simulink model "A_DIOL_BicopterControl"  (R2022a)
settings: Solver=FixedStepAuto  StartTime=0.0  StopTime=110  FixedStep=1e-4  RelTol=1e-3
values from neighbouring files (symbols this model uses):
  k = place(A,B,p)    [A_DIOL_runner.m]    (also in A_DIOL_sim_runner.m; print_DE_FL.m)
undefined symbols (not defined in the file or in its folder): sigbuilder_block
libraries: spsFirstOrderFilterLib x6
settings Model: Creator=PhDstudent1  LastModifiedBy=NITRO5

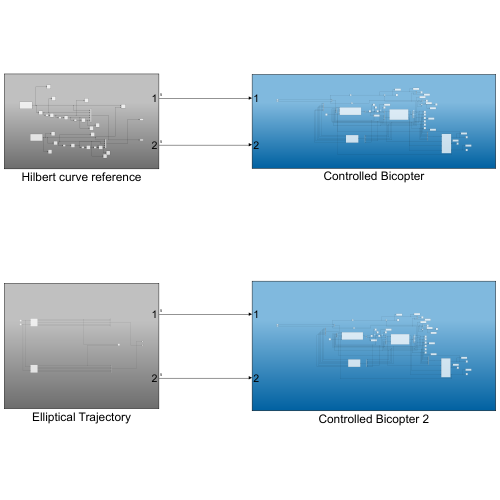
[thumbnail: Simulink's stored preview of the top-level diagram]
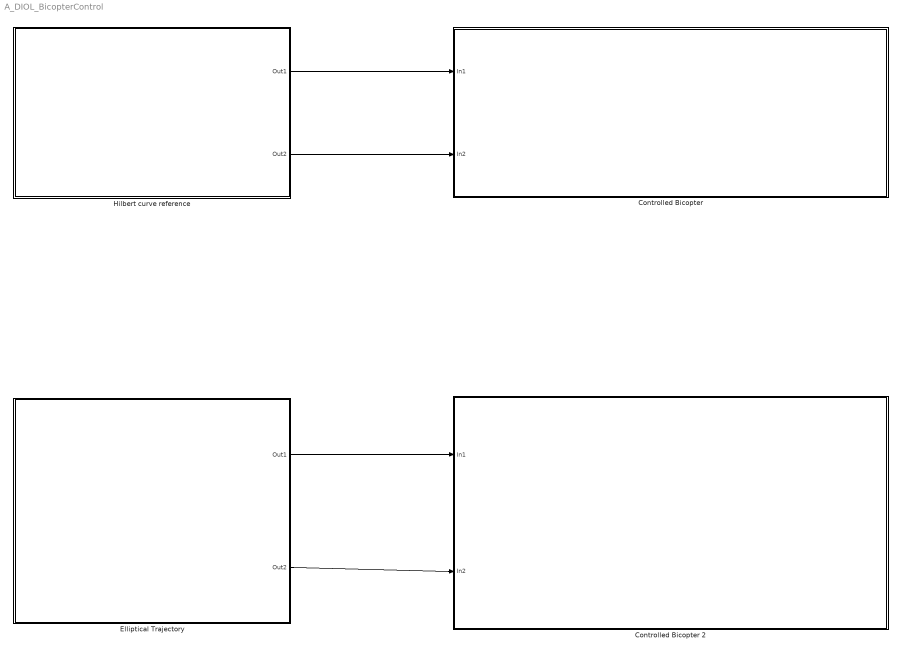
== system A_DIOL_BicopterControl ==
  Controlled Bicopter : Subsystem
  Controlled Bicopter 2 : Subsystem
  Elliptical Trajectory : Subsystem
  Hilbert curve reference : Subsystem
  wires:
  Hilbert curve reference/1(Out1) -> Controlled Bicopter/1(In1)
  Hilbert curve reference/2(Out2) -> Controlled Bicopter/2(In2)
  Elliptical Trajectory/1(Out1) -> Controlled Bicopter 2/1(In1)
  Elliptical Trajectory/2(Out2) -> Controlled Bicopter 2/2(In2)

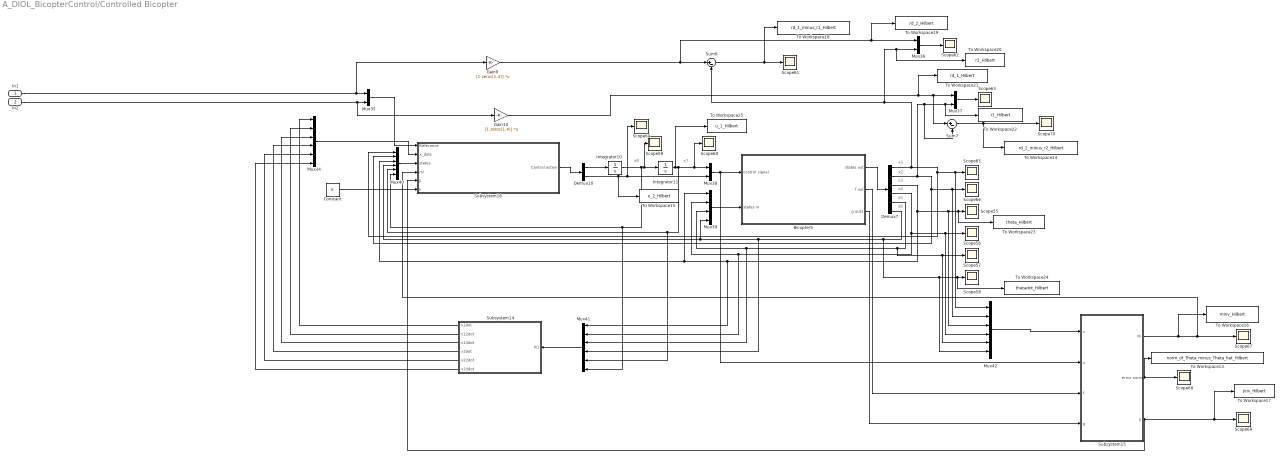
== system A_DIOL_BicopterControl/Controlled Bicopter ==
  note: x4
  note: x1
  note: x8
  note: x5
  note: x6
  note: x7
  note: x2
  note: x3
  In1 : Inport
  In2 : Inport  Port=2
  Bicopter5 : Subsystem
  Constant : Constant  Value=k
  Demux10 : Demux  Outputs=2
  Demux7 : Demux  Outputs=6
  Gain10 : Gain  Gain=[1 zeros(1,4)]  Multiplication=Matrix(K*u)
  Gain9 : Gain  Gain=[1 zeros(1,4)]  Multiplication=Matrix(K*u)
  Integrator10 : Integrator  InitialCondition=2
  Integrator11 : Integrator  InitialCondition=15
  Mux{34,40..42} (4 alike) : Mux  Inputs=6
  Mux{35..38} (4 alike) : Mux  Inputs=2
  Mux39 : Mux
  Scope{55..70} (16 alike) : Scope
  Subsystem14 : Subsystem
  Subsystem15 : Subsystem
  Subsystem16 : Subsystem
  Sum6 : Sum  Inputs=|+-
  Sum7 : Sum  Inputs=|+-
  To Workspace13 : ToWorkspace  VariableName=norm_of_Theta_minus_Theta_hat_Hilbert  SaveFormat=Timeseries  SampleTime=-1
  To Workspace14 : ToWorkspace  VariableName=rd_2_minus_r2_Hilbert  SaveFormat=Timeseries  SampleTime=-1
  To Workspace15 : ToWorkspace  VariableName=u_2_Hilbert  SaveFormat=Timeseries  SampleTime=-1
  To Workspace16 : ToWorkspace  VariableName=minv_Hilbert  SaveFormat=Timeseries  SampleTime=-1
  To Workspace17 : ToWorkspace  VariableName=Jinv_Hilbert  SaveFormat=Timeseries  SampleTime=-1
  To Workspace18 : ToWorkspace  VariableName=rd_1_minus_r1_Hilbert  SaveFormat=Timeseries  SampleTime=-1
  To Workspace19 : ToWorkspace  VariableName=rd_2_Hilbert  SaveFormat=Timeseries  SampleTime=-1
  To Workspace20 : ToWorkspace  VariableName=r2_Hilbert  SaveFormat=Timeseries  SampleTime=-1
  To Workspace21 : ToWorkspace  VariableName=rd_1_Hilbert  SaveFormat=Timeseries  SampleTime=-1
  To Workspace22 : ToWorkspace  VariableName=r1_Hilbert  SaveFormat=Timeseries  SampleTime=-1
  To Workspace23 : ToWorkspace  VariableName=theta_Hilbert  SaveFormat=Timeseries  SampleTime=-1
  To Workspace24 : ToWorkspace  VariableName=thetadot_Hilbert  SaveFormat=Timeseries  SampleTime=-1
  To Workspace25 : ToWorkspace  VariableName=u_1_Hilbert  SaveFormat=Timeseries  SampleTime=-1
  wires:
  Sum7/1 -> To Workspace14/1, Scope70/1
  Bicopter5/2(f out) -> Subsystem15/3(f)
  Demux7/6 -> Mux42/6, To Workspace24/1, Scope58/1, Mux41/4, Mux39/4, Mux40/4
  Demux7/2 -> Sum7/2, To Workspace22/1, Mux37/2, Mux42/2, Scope66/1, Mux40/2
  Demux7/1 -> To Workspace20/1, Mux36/2, Sum6/2, Mux42/1, Scope65/1, Mux40/1
  Subsystem14/6(x23dot) -> Mux34/6
  Demux7/4 -> Mux42/4, Scope56/1, Mux41/2, Mux39/2
  Bicopter5/1(states out) -> Demux7/1
  Integrator10/1 -> Mux41/6, Mux40/6, Scope59/1, Integrator11/1
  Mux42/1 -> Subsystem15/1(x)
  Subsystem15/2(error norm) -> To Workspace13/1, Scope68/1
  Demux7/5 -> Mux41/3, Mux39/3, Mux42/5, Scope57/1
  Mux39/1 -> Bicopter5/2(states in)
  Subsystem15/1(mi) -> To Workspace16/1, Scope67/1, Subsystem16/4(mi)
  Subsystem14/4(x2dot) -> Mux34/4
  Subsystem14/1(x1dot) -> Mux34/1
  Integrator11/1 -> To Workspace25/1, Mux41/5, Mux40/5, Scope60/1, Mux38/1
  Bicopter5/3(g out1) -> Subsystem15/4(g)
  Demux10/2 -> To Workspace15/1, Scope64/1, Mux38/2
  In2/1 -> Gain10/1, Mux35/2
  Gain9/1 -> To Workspace19/1, Mux36/1, Sum6/1
  Demux10/1 -> Integrator10/1
  Mux40/1 -> Subsystem16/3(states)
  In1/1 -> Gain9/1, Mux35/1
  Mux37/1 -> Scope63/1
  Subsystem15/3(Ji) -> Subsystem16/5(Ji), To Workspace17/1, Scope69/1
  Mux34/1 -> Subsystem16/2(x_dots)
  Subsystem16/1(Control action) -> Demux10/1
  Mux35/1 -> Subsystem16/1(Reference)
  Sum6/1 -> To Workspace18/1, Scope61/1
  Constant/1 -> Subsystem16/6(k)
  Subsystem14/2(x12dot) -> Mux34/2
  Gain10/1 -> To Workspace21/1, Sum7/1, Mux37/1
  Mux38/1 -> Subsystem15/2(u), Bicopter5/1(control signal)
  Demux7/3 -> Mux42/3, To Workspace23/1, Scope55/1, Mux41/1, Mux39/1, Mux40/3
  Mux41/1 -> Subsystem14/1(In1)
  Subsystem14/3(x13dot) -> Mux34/3
  Subsystem14/5(x22dot) -> Mux34/5
  Mux36/1 -> Scope62/1

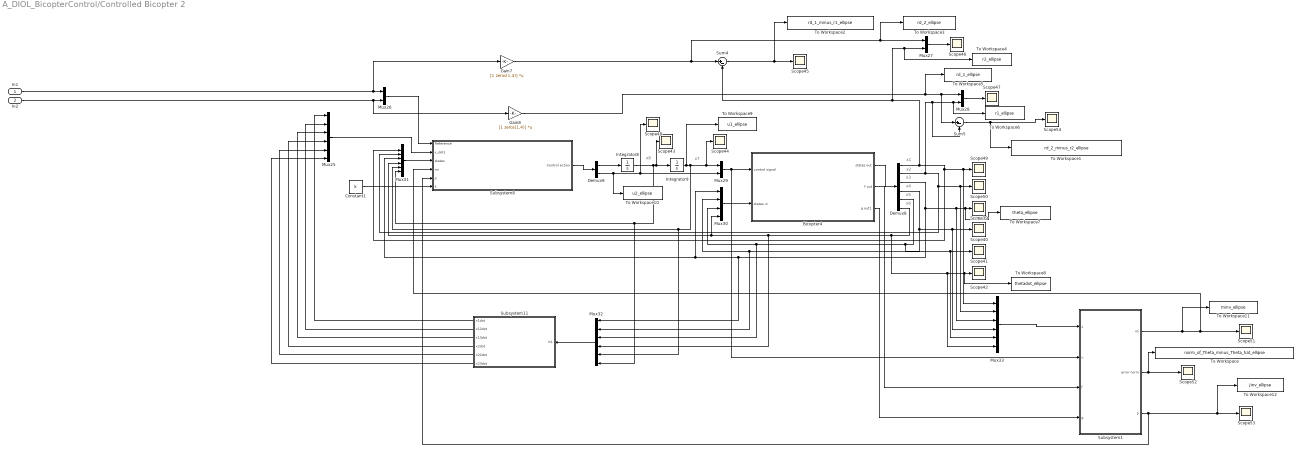
== system A_DIOL_BicopterControl/Controlled Bicopter 2 ==
  note: x4
  note: x1
  note: x8
  note: x6
  note: x5
  note: x7
  note: x3
  note: x2
  In1 : Inport
  In2 : Inport  Port=2
  Bicopter4 : Subsystem
  Constant1 : Constant  Value=k
  Demux8 : Demux  Outputs=6
  Demux9 : Demux  Outputs=2
  Gain7 : Gain  Gain=[1 zeros(1,4)]  Multiplication=Matrix(K*u)
  Gain8 : Gain  Gain=[1 zeros(1,4)]  Multiplication=Matrix(K*u)
  Integrator8 : Integrator
  Integrator9 : Integrator  InitialCondition=10
  Mux{25,31..33} (4 alike) : Mux  Inputs=6
  Mux{26..29} (4 alike) : Mux  Inputs=2
  Mux30 : Mux
  Scope{39..54} (16 alike) : Scope
  Subsystem1 : Subsystem
  Subsystem11 : Subsystem
  Subsystem8 : Subsystem
  Sum4 : Sum  Inputs=|+-
  Sum5 : Sum  Inputs=|+-
  To Workspace : ToWorkspace  VariableName=norm_of_Theta_minus_Theta_hat_ellipse  SaveFormat=Timeseries  SampleTime=-1
  To Workspace1 : ToWorkspace  VariableName=rd_2_minus_r2_ellipse  SaveFormat=Timeseries  SampleTime=-1
  To Workspace10 : ToWorkspace  VariableName=u2_ellipse  SaveFormat=Timeseries  SampleTime=-1
  To Workspace11 : ToWorkspace  VariableName=minv_ellipse  SaveFormat=Timeseries  SampleTime=-1
  To Workspace12 : ToWorkspace  VariableName=Jinv_ellipse  SaveFormat=Timeseries  SampleTime=-1
  To Workspace2 : ToWorkspace  VariableName=rd_1_minus_r1_ellipse  SaveFormat=Timeseries  SampleTime=-1
  To Workspace3 : ToWorkspace  VariableName=rd_2_ellipse  SaveFormat=Timeseries  SampleTime=-1
  To Workspace4 : ToWorkspace  VariableName=r2_ellipse  SaveFormat=Timeseries  SampleTime=-1
  To Workspace5 : ToWorkspace  VariableName=rd_1_ellipse  SaveFormat=Timeseries  SampleTime=-1
  To Workspace6 : ToWorkspace  VariableName=r1_ellipse  SaveFormat=Timeseries  SampleTime=-1
  To Workspace7 : ToWorkspace  VariableName=theta_ellipse  SaveFormat=Timeseries  SampleTime=-1
  To Workspace8 : ToWorkspace  VariableName=thetadot_ellipse  SaveFormat=Timeseries  SampleTime=-1
  To Workspace9 : ToWorkspace  VariableName=u1_ellipse  SaveFormat=Timeseries  SampleTime=-1
  wires:
  Subsystem11/2(x12dot) -> Mux25/2
  Demux8/6 -> Mux33/6, To Workspace8/1, Scope42/1, Mux32/4, Mux30/4, Mux31/4
  Subsystem1/3(Ji) -> To Workspace12/1, Scope53/1, Subsystem8/5(Ji)
  Integrator8/1 -> Mux32/6, Mux31/6, Scope43/1, Integrator9/1
  Subsystem11/6(x23dot) -> Mux25/6
  Demux8/4 -> Mux33/4, Scope40/1, Mux32/2, Mux30/2
  Integrator9/1 -> To Workspace9/1, Mux32/5, Mux31/5, Scope44/1, Mux29/1
  Demux8/1 -> To Workspace4/1, Mux27/2, Sum4/2, Mux33/1, Scope49/1, Mux31/1
  Subsystem1/1(mi) -> To Workspace11/1, Scope51/1, Subsystem8/4(mi)
  In1/1 -> Gain7/1, Mux26/1
  Demux8/2 -> Sum5/2, To Workspace6/1, Mux28/2, Mux33/2, Scope50/1, Mux31/2
  Subsystem8/1(Control action) -> Demux9/1
  Constant1/1 -> Subsystem8/6(k)
  Demux8/5 -> Mux32/3, Mux30/3, Mux33/5, Scope41/1
  Bicopter4/2(f out) -> Subsystem1/3(f)
  Subsystem11/5(x22dot) -> Mux25/5
  Subsystem11/3(x13dot) -> Mux25/3
  Mux27/1 -> Scope46/1
  Subsystem11/4(x2dot) -> Mux25/4
  Demux9/2 -> To Workspace10/1, Scope48/1, Mux29/2
  Demux9/1 -> Integrator8/1
  Mux26/1 -> Subsystem8/1(Reference)
  Mux30/1 -> Bicopter4/2(states in)
  Demux8/3 -> Mux33/3, To Workspace7/1, Scope39/1, Mux32/1, Mux30/1, Mux31/3
  Mux25/1 -> Subsystem8/2(x_dots)
  Gain7/1 -> To Workspace3/1, Mux27/1, Sum4/1
  Mux31/1 -> Subsystem8/3(states)
  Bicopter4/3(g out1) -> Subsystem1/4(g)
  Mux33/1 -> Subsystem1/1(x)
  Subsystem1/2(error norm) -> To Workspace/1, Scope52/1
  Mux29/1 -> Subsystem1/2(u), Bicopter4/1(control signal)
  Sum4/1 -> To Workspace2/1, Scope45/1
  Mux28/1 -> Scope47/1
  Mux32/1 -> Subsystem11/1(In1)
  Subsystem11/1(x1dot) -> Mux25/1
  Sum5/1 -> To Workspace1/1, Scope54/1
  In2/1 -> Gain8/1, Mux26/2
  Gain8/1 -> To Workspace5/1, Sum5/1, Mux28/1
  Bicopter4/1(states out) -> Demux8/1

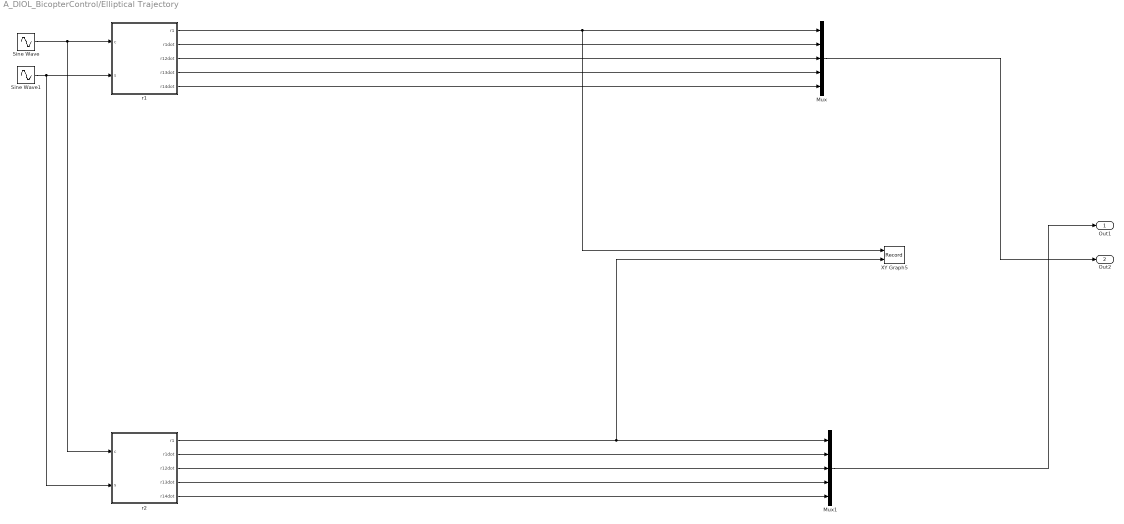
== system A_DIOL_BicopterControl/Elliptical Trajectory ==
  Mux : Mux  Inputs=5
  Mux1 : Mux  Inputs=5
  Sine Wave : Sin  Phase=pi/2  SampleTime=0
  Sine Wave1 : Sin  SampleTime=0
  XY Graph5 : Record  FileSettingsInternal="{\"entries\":[{\"content\":{\"excelSettings\":{\"content\":{},\"type\":\"Streamout.ExcelSettings\"}},\"type\":\"Streamout.FileSettingStorage\",\"uuid\":\"26a49ed7-52eb-4951-809f-6988e8d13940\"}],\"packageUris\":[\"http://schema.mathworks.com/mf0/streamout_blocks/R2020a\"],\"version\":\"1.0\"}"  Layout=[1 1]  SignalsInternal="{\"entries\":[{\"content\":{\"signals\":[{\"content\":{\"blockPath\":[\"DE_IOL/Elliptical Trajectory/XY Graph5\"],\"channel\":[],\"dimensions\":[1],\"domain\":\"DE_IOL/Elliptical Trajectory/XY Graph5\",\"lineColor\":\"#0072bd\",\"plots\":[],\"port\":1,\"sid\":[],\"signalID\":8873,\"signalName\":\"r1:1\"},\"type\":\"RecordBlkView.Signal\",\"uuid\":\"5bdcea52-0e7e-48eb-8d84-bb9175bf30af\"},{\"content\":{\"blockPath\":[\"DE_IOL/Elliptical Trajectory/XY Graph5\"],\"channel\":[],\"dimensions\":[1],\"domain\":\"DE_IOL/Elliptical Trajectory/XY Graph5\",\"lineColor\":\"#d95319\",\"plots\":[],\"port\":2,\"sid\":[],\"signalID\":8876,\"signalName\":\"r2:1\"},\"type\":\"RecordBlkView.Signal\",\"uuid\":\"504f0850-e16c-4121-9ee7-25123b3e2c1d\"}]},\"type\":\"RecordBlkView.InputSignals\",\"uuid\":\"3da81941-7f27-4a40-ba46-ff9135730fe0\"}],\"packageUris\":[\"http://schema.mathworks.com/mf0/streamout_blocks/R2020a\"],\"version\":\"1.0\"}"  VisualizationBindings="{\"xyplotplugin\":{\"info\":[{\"series\":[],\"subplotID\":1}]}}"  CompatibilityTag=XY
  r1 : MATLAB Function  TreatAsAtomicUnit=on
  r2 : MATLAB Function  TreatAsAtomicUnit=on
  Out1 : Outport
  Out2 : Outport  Port=2
  wires:
  Mux/1 -> Out2/1
  Mux1/1 -> Out1/1
  Sine Wave/1 -> r2/1(c), r1/1(c)
  Sine Wave1/1 -> r2/2(s), r1/2(s)
  r1/1(r1) -> XY Graph5/1, Mux/1
  r1/2(r1dot) -> Mux/2
  r1/3(r12dot) -> Mux/3
  r1/4(r13dot) -> Mux/4
  r1/5(r14dot) -> Mux/5
  r2/1(r1) -> XY Graph5/2, Mux1/1
  r2/2(r1dot) -> Mux1/2
  r2/3(r12dot) -> Mux1/3
  r2/4(r13dot) -> Mux1/4
  r2/5(r14dot) -> Mux1/5

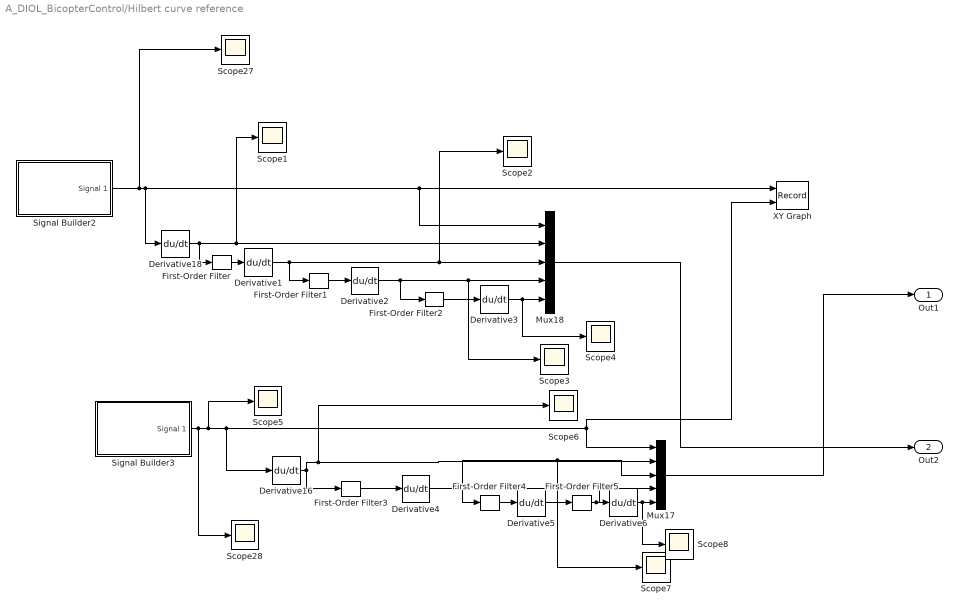
== system A_DIOL_BicopterControl/Hilbert curve reference ==
  Derivative{1..6,16,18} (8 alike) : Derivative
  First-Order Filter{,1..5} (6 alike) : spsFirstOrderFilterLib/First-Order Filter  FilterType=Lowpass  Tc=5e-01  Ts=0  Initialize=on  Vac_Init=[0, 0, 60]  Vdc_Init=0  PlotResponse=off  FreqRange="[0,  200,  1]"
  Mux17 : Mux  Inputs=5
  Mux18 : Mux  Inputs=5
  Scope{1..8,27..28} (10 alike) : Scope
  Signal Builder2 : Subsystem  Tag=STV Subsys  LoadFcn=sigbuilder_block('load');  StartFcn=sigbuilder_block('start');  StopFcn=sigbuilder_block('stop');  ClipboardFcn=sigbuilder_block('clipboard');  mask(Sigbuilder block){tuvar=[0:10]}
      mask help: Simulink:masks:SigbuilderBlock_MD
      mask init:
      | if ~strcmp(get_param(bdroot(gcbh),'SimulationStatus'),'stopped') tuvar = sigbuilder_block('maskInit'); end
      settings: CopyFcn=sigbuilder_block('copy');  DeleteFcn=sigbuilder_block('delete');  ModelCloseFcn=sigbuilder_block('modelClose');  PreSaveFcn=sigbuilder_block('preSave');  PauseFcn=sigbuilder_block('pause');  ContinueFcn=sigbuilder_block('continue');  NameChangeFcn=sigbuilder_block('namechange');  OpenFcn=sigbuilder_block('open',[438.6 146.4 550.8 400.2 ]);  CloseFcn=sigbuilder_block('close');
      mask Display: plot(0, 0, 100, 100,[2, 2, 32, 32, 2], [68, 8, 8, 68, 68],[32, 2], [38, 38], [32, 19, 2],[53, 60, 44], [32, 17, 17, 2],[16, 16, 31, 31]);txt = getActiveGroup(gcbh);text(2, 100, txt,'verticalAlignment', 'top');
  Signal Builder3 : Subsystem  Tag=STV Subsys  LoadFcn=sigbuilder_block('load');  StartFcn=sigbuilder_block('start');  StopFcn=sigbuilder_block('stop');  ClipboardFcn=sigbuilder_block('clipboard');  mask(Sigbuilder block){tuvar=[0:10]}
      mask help: Simulink:masks:SigbuilderBlock_MD
      mask init:
      | if ~strcmp(get_param(bdroot(gcbh),'SimulationStatus'),'stopped') tuvar = sigbuilder_block('maskInit'); end
      settings: CopyFcn=sigbuilder_block('copy');  DeleteFcn=sigbuilder_block('delete');  ModelCloseFcn=sigbuilder_block('modelClose');  PreSaveFcn=sigbuilder_block('preSave');  PauseFcn=sigbuilder_block('pause');  ContinueFcn=sigbuilder_block('continue');  NameChangeFcn=sigbuilder_block('namechange');  OpenFcn=sigbuilder_block('open',[437.6 199.2 550.4 400 ]);  CloseFcn=sigbuilder_block('close');
      mask Display: plot(0, 0, 100, 100,[2, 2, 32, 32, 2], [68, 8, 8, 68, 68],[32, 2], [38, 38], [32, 19, 2],[53, 60, 44], [32, 17, 17, 2],[16, 16, 31, 31]);txt = getActiveGroup(gcbh);text(2, 100, txt,'verticalAlignment', 'top');
  XY Graph : Record  FileSettingsInternal="{\"entries\":[{\"content\":{\"excelSettings\":{\"content\":{},\"type\":\"Streamout.ExcelSettings\"}},\"type\":\"Streamout.FileSettingStorage\",\"uuid\":\"b2cb4743-b414-4fa3-b39c-92ceac2c3444\"}],\"packageUris\":[\"http://schema.mathworks.com/mf0/streamout_blocks/R2020a\"],\"version\":\"1.0\"}"  Layout=[1 1]  SignalsInternal="{\"entries\":[{\"content\":{\"signals\":[{\"content\":{\"blockPath\":[\"DE_IOL/Hilbert curve reference/XY Graph\"],\"channel\":[],\"dimensions\":[1],\"domain\":\"DE_IOL/Hilbert curve reference/XY Graph\",\"lineColor\":\"#22b573\",\"plots\":[],\"port\":1,\"sid\":[],\"signalID\":8865,\"signalName\":\"Signal Builder2\"},\"type\":\"RecordBlkView.Signal\",\"uuid\":\"2da99c1a-afef-41a8-b7fd-2517c81241d1\"},{\"content\":{\"blockPath\":[\"DE_IOL/Hilbert curve reference/XY Graph\"],\"channel\":[],\"dimensions\":[1],\"domain\":\"DE_IOL/Hilbert curve reference/XY Graph\",\"lineColor\":\"#0072bd\",\"plots\":[],\"port\":2,\"sid\":[],\"signalID\":8868,\"signalName\":\"Signal Builder3\"},\"type\":\"RecordBlkView.Signal\",\"uuid\":\"8f8a0f8d-85d2-41e9-a624-d09f38dfe041\"}]},\"type\":\"RecordBlkView.InputSignals\",\"uuid\":\"13dae95f-34ba-4b2e-9c06-6b2fd417d590\"}],\"packageUris\":[\"http://schema.mathworks.com/mf0/streamout_blocks/R2020a\"],\"version\":\"1.0\"}"  VisualizationBindings="{\"xyplotplugin\":{\"info\":[{\"series\":[],\"subplotID\":1}]}}"  CompatibilityTag=XY
  Out1 : Outport
  Out2 : Outport  Port=2
  wires:
  Signal Builder2/1(Signal 1) -> Scope27/1, Mux18/1, XY Graph/1, Derivative18/1
  Derivative16/1 -> First-Order Filter3/1, Scope6/1, Mux17/2
  Signal Builder3/1(Signal 1) -> Scope28/1, Scope5/1, Derivative16/1, XY Graph/2, Mux17/1
  Mux17/1 -> Out1/1
  Mux18/1 -> Out2/1
  Derivative1/1 -> Scope2/1, Mux18/3, First-Order Filter1/1
  Derivative2/1 -> Scope3/1, Mux18/4, First-Order Filter2/1
  Derivative3/1 -> Scope4/1, Mux18/5
  Derivative4/1 -> First-Order Filter4/1, Scope7/1, Mux17/3
  Derivative5/1 -> First-Order Filter5/1
  Derivative6/1 -> Scope8/1, Mux17/5
  Derivative18/1 -> Scope1/1, Mux18/2, First-Order Filter/1
  First-Order Filter/1 -> Derivative1/1
  First-Order Filter1/1 -> Derivative2/1
  First-Order Filter2/1 -> Derivative3/1
  First-Order Filter3/1 -> Derivative4/1
  First-Order Filter4/1 -> Derivative5/1
  First-Order Filter5/1 -> Mux17/4, Derivative6/1

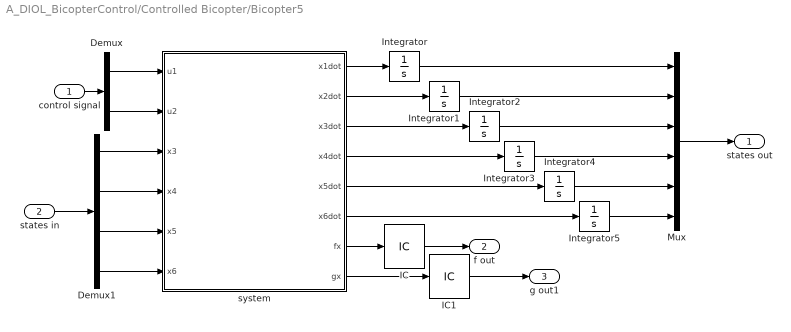
== system A_DIOL_BicopterControl/Controlled Bicopter/Bicopter5 ==
  control signal : Inport
  states in : Inport  Port=2
  Demux : Demux  Outputs=2
  Demux1 : Demux
  IC : InitialCondition  Value=zeros(6,1)
  IC1 : InitialCondition  Value=zeros(6,2)
  Integrator : Integrator  InitialCondition=0.01
  Integrator1 : Integrator
  Integrator2 : Integrator  InitialCondition=0.03
  Integrator3 : Integrator  InitialCondition=0.02
  Integrator4 : Integrator  InitialCondition=0.01
  Integrator5 : Integrator
  Mux : Mux  Inputs=6
  system : MATLAB Function  TreatAsAtomicUnit=on
  states out : Outport
  f out : Outport  Port=2
  g out1 : Outport  Port=3
  wires:
  Integrator5/1 -> Mux/6
  system/2(x2dot) -> Integrator1/1
  Integrator/1 -> Mux/1
  Integrator4/1 -> Mux/5
  system/6(x6dot) -> Integrator5/1
  Integrator3/1 -> Mux/4
  Integrator1/1 -> Mux/2
  system/1(x1dot) -> Integrator/1
  Demux/1 -> system/1(u1)
  system/4(x4dot) -> Integrator3/1
  system/5(x5dot) -> Integrator4/1
  Demux1/2 -> system/4(x4)
  Demux1/4 -> system/6(x6)
  Demux1/3 -> system/5(x5)
  system/3(x3dot) -> Integrator2/1
  Demux/2 -> system/2(u2)
  Demux1/1 -> system/3(x3)
  Integrator2/1 -> Mux/3
  control signal/1 -> Demux/1
  Mux/1 -> states out/1
  states in/1 -> Demux1/1
  system/7(fx) -> IC/1
  system/8(gx) -> IC1/1
  IC/1 -> f out/1
  IC1/1 -> g out1/1

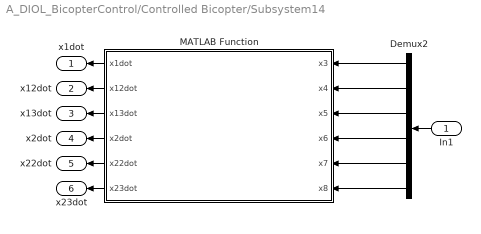
== system A_DIOL_BicopterControl/Controlled Bicopter/Subsystem14 ==
  In1 : Inport
  Demux2 : Demux  Outputs=6
  MATLAB Function : MATLAB Function  TreatAsAtomicUnit=on
  x1dot : Outport
  x12dot : Outport  Port=2
  x13dot : Outport  Port=3
  x2dot : Outport  Port=4
  x22dot : Outport  Port=5
  x23dot : Outport  Port=6
  wires:
  Demux2/3 -> MATLAB Function/3(x5)
  MATLAB Function/5(x22dot) -> x22dot/1
  Demux2/6 -> MATLAB Function/6(x8)
  Demux2/1 -> MATLAB Function/1(x3)
  Demux2/2 -> MATLAB Function/2(x4)
  Demux2/4 -> MATLAB Function/4(x6)
  Demux2/5 -> MATLAB Function/5(x7)
  MATLAB Function/4(x2dot) -> x2dot/1
  MATLAB Function/6(x23dot) -> x23dot/1
  In1/1 -> Demux2/1
  MATLAB Function/3(x13dot) -> x13dot/1
  MATLAB Function/1(x1dot) -> x1dot/1
  MATLAB Function/2(x12dot) -> x12dot/1

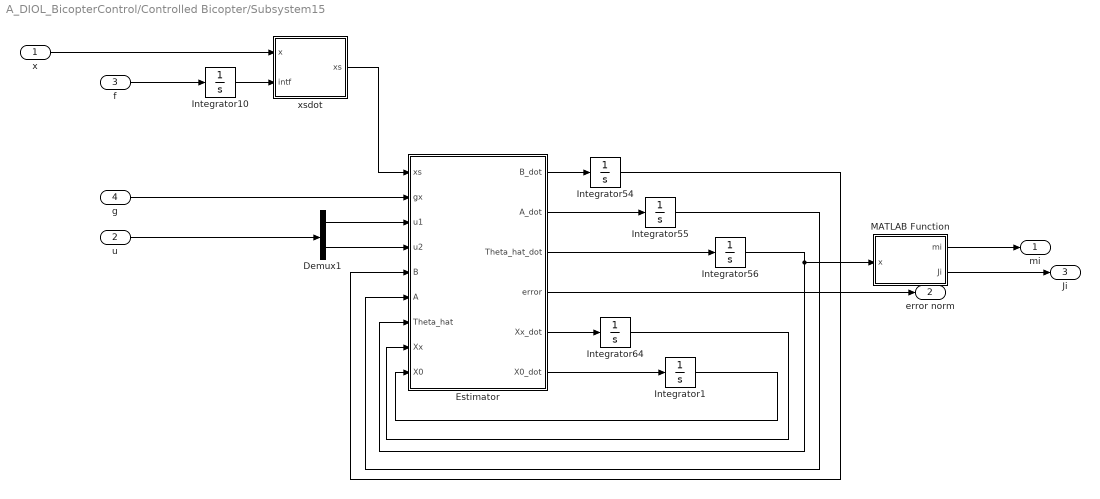
== system A_DIOL_BicopterControl/Controlled Bicopter/Subsystem15 ==
  x : Inport
  u : Inport  Port=2
  f : Inport  Port=3
  g : Inport  Port=4
  Demux1 : Demux  Outputs=2
  Estimator : MATLAB Function  TreatAsAtomicUnit=on
  Integrator1 : Integrator  InitialCondition=zeros(6,2)
  Integrator10 : Integrator  InitialCondition=[0;0;0;0;0;0]
  Integrator54 : Integrator  InitialCondition=ones(2,2)
  Integrator55 : Integrator
  Integrator56 : Integrator  InitialCondition=[2 10]
  Integrator64 : Integrator
  MATLAB Function : MATLAB Function  TreatAsAtomicUnit=on
  xsdot : MATLAB Function  TreatAsAtomicUnit=on
  mi : Outport
  error norm : Outport  Port=2
  Ji : Outport  Port=3
  wires:
  Integrator10/1 -> xsdot/2(intf)
  xsdot/1(xs) -> Estimator/1(xs)
  Demux1/1 -> Estimator/3(u1)
  Demux1/2 -> Estimator/4(u2)
  Estimator/1(B_dot) -> Integrator54/1
  Estimator/2(A_dot) -> Integrator55/1
  Estimator/3(Theta_hat_dot) -> Integrator56/1
  Integrator54/1 -> Estimator/5(B)
  Integrator55/1 -> Estimator/6(A)
  Integrator56/1 -> MATLAB Function/1(x), Estimator/7(Theta_hat)
  Estimator/4(error) -> error norm/1
  Estimator/5(Xx_dot) -> Integrator64/1
  Estimator/6(X0_dot) -> Integrator1/1
  Integrator64/1 -> Estimator/8(Xx)
  Integrator1/1 -> Estimator/9(X0)
  u/1 -> Demux1/1
  MATLAB Function/1(mi) -> mi/1
  f/1 -> Integrator10/1
  g/1 -> Estimator/2(gx)
  x/1 -> xsdot/1(x)
  MATLAB Function/2(Ji) -> Ji/1

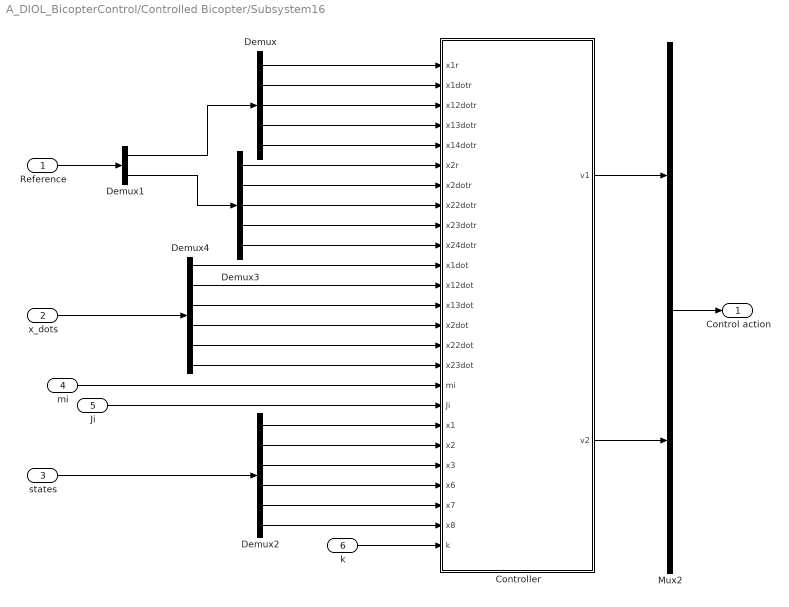
== system A_DIOL_BicopterControl/Controlled Bicopter/Subsystem16 ==
  Reference : Inport
  x_dots : Inport  Port=2
  states : Inport  Port=3
  mi : Inport  Port=4
  Ji : Inport  Port=5
  k : Inport  Port=6
  Controller : MATLAB Function  TreatAsAtomicUnit=on
  Demux : Demux  Outputs=5
  Demux1 : Demux  Outputs=2
  Demux2 : Demux  Outputs=6
  Demux3 : Demux  Outputs=5
  Demux4 : Demux  Outputs=6
  Mux2 : Mux  Inputs=2
  Control action : Outport
  wires:
  Demux2/2 -> Controller/20(x2)
  Controller/2(v2) -> Mux2/2
  Demux2/6 -> Controller/24(x8)
  Demux2/5 -> Controller/23(x7)
  Demux2/4 -> Controller/22(x6)
  Controller/1(v1) -> Mux2/1
  Demux2/3 -> Controller/21(x3)
  Demux2/1 -> Controller/19(x1)
  Reference/1 -> Demux1/1
  Mux2/1 -> Control action/1
  Demux/1 -> Controller/1(x1r)
  Demux/2 -> Controller/2(x1dotr)
  Demux/3 -> Controller/3(x12dotr)
  Demux/4 -> Controller/4(x13dotr)
  Demux/5 -> Controller/5(x14dotr)
  Demux3/2 -> Controller/7(x2dotr)
  Demux3/3 -> Controller/8(x22dotr)
  Demux3/4 -> Controller/9(x23dotr)
  Demux3/5 -> Controller/10(x24dotr)
  Demux3/1 -> Controller/6(x2r)
  Demux1/1 -> Demux/1
  Demux1/2 -> Demux3/1
  Demux4/2 -> Controller/12(x12dot)
  Demux4/3 -> Controller/13(x13dot)
  Demux4/4 -> Controller/14(x2dot)
  Demux4/5 -> Controller/15(x22dot)
  Demux4/6 -> Controller/16(x23dot)
  Demux4/1 -> Controller/11(x1dot)
  x_dots/1 -> Demux4/1
  states/1 -> Demux2/1
  mi/1 -> Controller/17(mi)
  Ji/1 -> Controller/18(Ji)
  k/1 -> Controller/25(k)

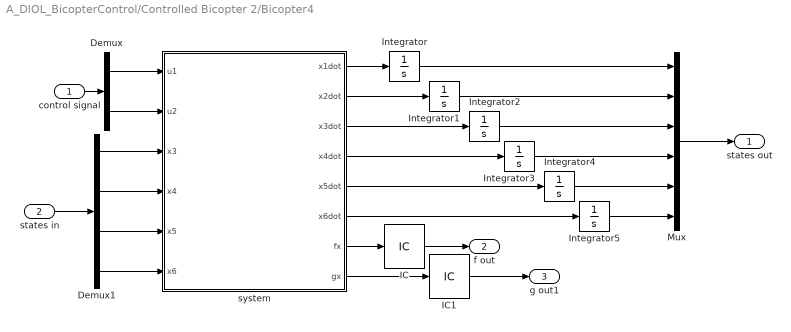
== system A_DIOL_BicopterControl/Controlled Bicopter 2/Bicopter4 ==
  control signal : Inport
  states in : Inport  Port=2
  Demux : Demux  Outputs=2
  Demux1 : Demux
  IC : InitialCondition  Value=zeros(6,1)
  IC1 : InitialCondition  Value=zeros(6,2)
  Integrator : Integrator  InitialCondition=0.01
  Integrator1 : Integrator  InitialCondition=0.02
  Integrator2 : Integrator  InitialCondition=0.03
  Integrator3 : Integrator  InitialCondition=0.02
  Integrator4 : Integrator  InitialCondition=0.01
  Integrator5 : Integrator
  Mux : Mux  Inputs=6
  system : MATLAB Function  TreatAsAtomicUnit=on
  states out : Outport
  f out : Outport  Port=2
  g out1 : Outport  Port=3
  wires:
  Integrator5/1 -> Mux/6
  system/2(x2dot) -> Integrator1/1
  Integrator/1 -> Mux/1
  Integrator4/1 -> Mux/5
  system/6(x6dot) -> Integrator5/1
  Integrator3/1 -> Mux/4
  Integrator1/1 -> Mux/2
  system/1(x1dot) -> Integrator/1
  Demux/1 -> system/1(u1)
  system/4(x4dot) -> Integrator3/1
  system/5(x5dot) -> Integrator4/1
  Demux1/2 -> system/4(x4)
  Demux1/4 -> system/6(x6)
  Demux1/3 -> system/5(x5)
  system/3(x3dot) -> Integrator2/1
  Demux/2 -> system/2(u2)
  Demux1/1 -> system/3(x3)
  Integrator2/1 -> Mux/3
  control signal/1 -> Demux/1
  Mux/1 -> states out/1
  states in/1 -> Demux1/1
  system/7(fx) -> IC/1
  system/8(gx) -> IC1/1
  IC/1 -> f out/1
  IC1/1 -> g out1/1

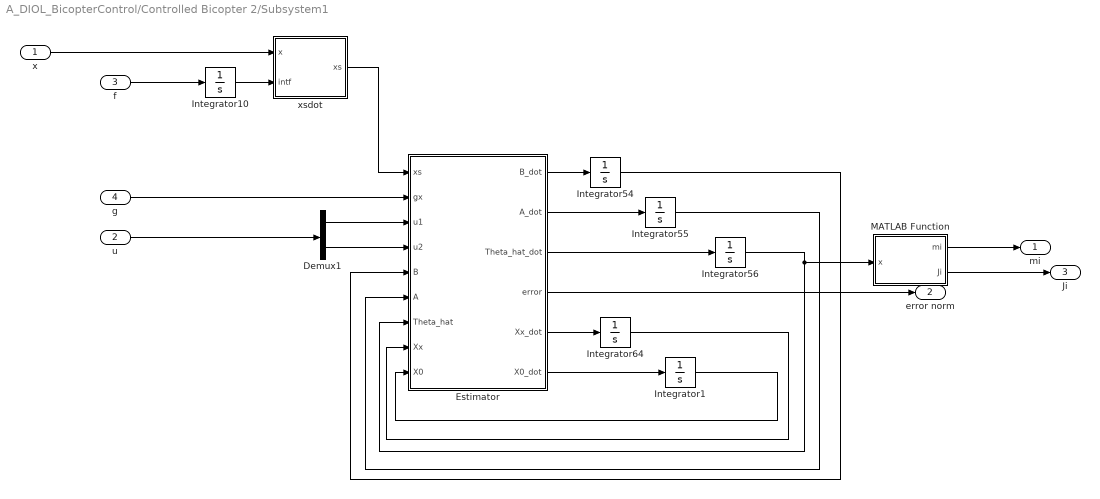
== system A_DIOL_BicopterControl/Controlled Bicopter 2/Subsystem1 ==
  x : Inport
  u : Inport  Port=2
  f : Inport  Port=3
  g : Inport  Port=4
  Demux1 : Demux  Outputs=2
  Estimator : MATLAB Function  TreatAsAtomicUnit=on
  Integrator1 : Integrator  InitialCondition=zeros(6,2)
  Integrator10 : Integrator  InitialCondition=[0;0;0;0;0;0]
  Integrator54 : Integrator  InitialCondition=ones(2,2)
  Integrator55 : Integrator
  Integrator56 : Integrator  InitialCondition=[2 10]
  Integrator64 : Integrator
  MATLAB Function : MATLAB Function  TreatAsAtomicUnit=on
  xsdot : MATLAB Function  TreatAsAtomicUnit=on
  mi : Outport
  error norm : Outport  Port=2
  Ji : Outport  Port=3
  wires:
  Integrator10/1 -> xsdot/2(intf)
  xsdot/1(xs) -> Estimator/1(xs)
  Demux1/1 -> Estimator/3(u1)
  Demux1/2 -> Estimator/4(u2)
  Estimator/1(B_dot) -> Integrator54/1
  Estimator/2(A_dot) -> Integrator55/1
  Estimator/3(Theta_hat_dot) -> Integrator56/1
  Integrator54/1 -> Estimator/5(B)
  Integrator55/1 -> Estimator/6(A)
  Integrator56/1 -> MATLAB Function/1(x), Estimator/7(Theta_hat)
  Estimator/4(error) -> error norm/1
  Estimator/5(Xx_dot) -> Integrator64/1
  Estimator/6(X0_dot) -> Integrator1/1
  Integrator64/1 -> Estimator/8(Xx)
  Integrator1/1 -> Estimator/9(X0)
  u/1 -> Demux1/1
  MATLAB Function/1(mi) -> mi/1
  f/1 -> Integrator10/1
  g/1 -> Estimator/2(gx)
  x/1 -> xsdot/1(x)
  MATLAB Function/2(Ji) -> Ji/1

== system A_DIOL_BicopterControl/Controlled Bicopter 2/Subsystem11 ==
  In1 : Inport
  Demux2 : Demux  Outputs=6
  MATLAB Function : MATLAB Function  TreatAsAtomicUnit=on
  x1dot : Outport
  x12dot : Outport  Port=2
  x13dot : Outport  Port=3
  x2dot : Outport  Port=4
  x22dot : Outport  Port=5
  x23dot : Outport  Port=6
  wires:
  Demux2/3 -> MATLAB Function/3(x5)
  MATLAB Function/5(x22dot) -> x22dot/1
  Demux2/6 -> MATLAB Function/6(x8)
  Demux2/1 -> MATLAB Function/1(x3)
  Demux2/2 -> MATLAB Function/2(x4)
  Demux2/4 -> MATLAB Function/4(x6)
  Demux2/5 -> MATLAB Function/5(x7)
  MATLAB Function/4(x2dot) -> x2dot/1
  MATLAB Function/6(x23dot) -> x23dot/1
  In1/1 -> Demux2/1
  MATLAB Function/3(x13dot) -> x13dot/1
  MATLAB Function/1(x1dot) -> x1dot/1
  MATLAB Function/2(x12dot) -> x12dot/1

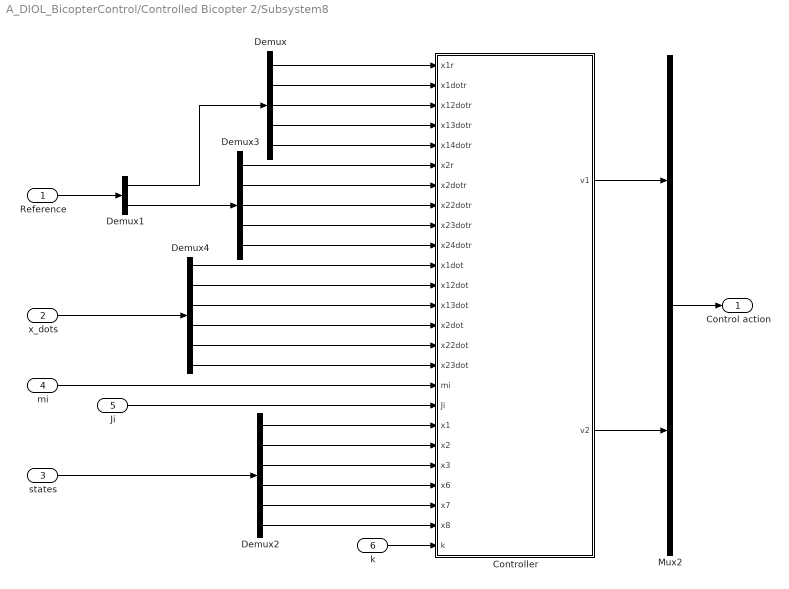
== system A_DIOL_BicopterControl/Controlled Bicopter 2/Subsystem8 ==
  Reference : Inport
  x_dots : Inport  Port=2
  states : Inport  Port=3
  mi : Inport  Port=4
  Ji : Inport  Port=5
  k : Inport  Port=6
  Controller : MATLAB Function  TreatAsAtomicUnit=on
  Demux : Demux  Outputs=5
  Demux1 : Demux  Outputs=2
  Demux2 : Demux  Outputs=6
  Demux3 : Demux  Outputs=5
  Demux4 : Demux  Outputs=6
  Mux2 : Mux  Inputs=2
  Control action : Outport
  wires:
  Demux2/2 -> Controller/20(x2)
  Controller/2(v2) -> Mux2/2
  Demux2/6 -> Controller/24(x8)
  Demux2/5 -> Controller/23(x7)
  Demux2/4 -> Controller/22(x6)
  Controller/1(v1) -> Mux2/1
  Demux2/3 -> Controller/21(x3)
  Demux2/1 -> Controller/19(x1)
  Reference/1 -> Demux1/1
  Mux2/1 -> Control action/1
  Demux/1 -> Controller/1(x1r)
  Demux/2 -> Controller/2(x1dotr)
  Demux/3 -> Controller/3(x12dotr)
  Demux/4 -> Controller/4(x13dotr)
  Demux/5 -> Controller/5(x14dotr)
  Demux3/2 -> Controller/7(x2dotr)
  Demux3/3 -> Controller/8(x22dotr)
  Demux3/4 -> Controller/9(x23dotr)
  Demux3/5 -> Controller/10(x24dotr)
  Demux3/1 -> Controller/6(x2r)
  Demux1/1 -> Demux/1
  Demux1/2 -> Demux3/1
  Demux4/2 -> Controller/12(x12dot)
  Demux4/3 -> Controller/13(x13dot)
  Demux4/4 -> Controller/14(x2dot)
  Demux4/5 -> Controller/15(x22dot)
  Demux4/6 -> Controller/16(x23dot)
  Demux4/1 -> Controller/11(x1dot)
  x_dots/1 -> Demux4/1
  states/1 -> Demux2/1
  mi/1 -> Controller/17(mi)
  Ji/1 -> Controller/18(Ji)
  k/1 -> Controller/25(k)

== system A_DIOL_BicopterControl/Hilbert curve reference/Signal Builder2 ==
  Demux : Demux  Tag=STV Demux  Outputs=1
      settings: DisplayOption=none
  FromWs : FromWorkspace  Tag=STV FromWs  VariableName=tuvar
      SigBuilderData=|
      | common.afterFinalStr = 'Extrapolate'
      | common.sampleTime = 0
      | dataSet.timeRange = [0 110]
      | dataSet.name = 'Group 1'
      | sbobj.Groups.Name = 'Group 1'
      | sbobj.Groups.Signals.Name = 'Signal 1'
      | sbobj.Groups.Signals.XData = [0 7 14 21 35 42 49 56 65 70 84 91 98 105 110]
      | sbobj.Groups.Signals.YData = [0 4 4 0 0 4 4 8 8 12 12 8 8 12 12]
      | sbobj.Groups.TimeRange = [0 110]
  Signal 1 : Outport  Tag=STV Outport
  wires:
  Demux/1 -> Signal 1/1
  FromWs/1 -> Demux/1

== system A_DIOL_BicopterControl/Hilbert curve reference/Signal Builder3 ==
  Demux : Demux  Tag=STV Demux  Outputs=1
      settings: DisplayOption=none
  FromWs : FromWorkspace  Tag=STV FromWs  VariableName=tuvar
      SigBuilderData=|
      | common.afterFinalStr = 'Extrapolate'
      | common.sampleTime = 0
      | dataSet.timeRange = [0 110]
      | dataSet.name = 'Group 1'
      | sbobj.Groups.Name = 'Group 1'
      | sbobj.Groups.Signals.Name = 'Signal 1'
      | sbobj.Groups.Signals.XData = [0 7 14 21 35 42 49 56 63 70 84 91 98 105 110]
      | sbobj.Groups.Signals.YData = [0 0 -7 -7 -21 -21 -14 -14 -21 -21 -7 -7 0 0 0]
      | sbobj.Groups.TimeRange = [0 110]
  Signal 1 : Outport  Tag=STV Outport
  wires:
  Demux/1 -> Signal 1/1
  FromWs/1 -> Demux/1

== matlab function A_DIOL_BicopterControl/Controlled Bicopter 2/Subsystem8/Controller ==
  data: x1r input; x1dotr input; x12dotr input; x13dotr input; x14dotr input; v1 output; x2r input; x2dotr input; x22dotr input; x23dotr input; x24dotr input; x1dot input; x12dot input; x13dot input; x2dot input; x22dot input; x23dot input; mi input; Ji input; x1 input; x2 input; x3 input; x6 input; x7 input; x8 input; v2 output; k input
function [v1,v2] = fcn(x1r,x1dotr,x12dotr,x13dotr,x14dotr,x2r,x2dotr,x22dotr,x23dotr,x24dotr,x1dot,x12dot,x13dot,x2dot,x22dot,x23dot,mi,Ji,x1,x2,x3,x6,x7,x8,k)

m = 1/mi;
J = 1/Ji;

% m = 1;
% J = 1;
% k1 = 19;
% k2 = 134.75;
% k3 = 422.75;
% k4 = 495;
% 
% k5 = 19;
% k6 = 134.75;
% k7 = 422.75;
% k8 = 495;
% 
% 
% 
% v1 = x7*x6^2 - m*cos(x3)*(k6*(x22dot - x22dotr) - x24dotr + k5*(x23dot - x23dotr) ...
%     + k8*(x2 - x2r) + k7*(x2dot - x2dotr)) + m*sin(x3)*(k2*(x12dot - x12dotr) - x14dotr + k1*(x13dot - x13dotr) + k4*(x1 - x1r) + k3*(x1dot - x1dotr));
% v2 = (J*m*cos(x3)*(k2*(x12dot - x12dotr) - x14dotr + k1*(x13dot - x13dotr) ...
%     + k4*(x1 - x1r) + k3*(x1dot - x1dotr)))/x7 - (2*J*x6*x8)/x7 + (J*m*sin(x3)*(k6*(x22dot - x22dotr) - x24dotr + k5*(x23dot - x23dotr) + k8*(x2 - x2r) + k7*(x2dot - x2dotr)))/x7;

k4 = k(1,4);
k3 = k(1,3);
k2 = k(1,2);
k1 = k(1,1);

k8 = k(2,8);
k7 = k(2,7);
k6 = k(2,6);
k5 = k(2,5);


v1 = x7*x6^2 - m*cos(x3)*(k7*(x22dot - x22dotr) - x24dotr + k8*(x23dot - x23dotr) ...
    + k5*(x2 - x2r) + k6*(x2dot - x2dotr)) + m*sin(x3)*(k3*(x12dot - x12dotr) - x14dotr ...
    + k4*(x13dot - x13dotr) + k1*(x1 - x1r) + k2*(x1dot - x1dotr));
v2 = (J*m*cos(x3)*(k3*(x12dot - x12dotr) - x14dotr + k4*(x13dot - x13dotr) ...
    + k1*(x1 - x1r) + k2*(x1dot - x1dotr)))/x7 - (2*J*x6*x8)/x7 ...
    + (J*m*sin(x3)*(k7*(x22dot - x22dotr) - x24dotr + k8*(x23dot - x23dotr) ...
    + k5*(x2 - x2r) + k6*(x2dot - x2dotr)))/x7;

end

== matlab function A_DIOL_BicopterControl/Controlled Bicopter/Bicopter5/system ==
  data: u1 input; x1dot output; u2 input; x3 input; x4 input; x5 input; x6 input; x2dot output; x3dot output; x4dot output; x5dot output; x6dot output; fx output; gx output
function [x1dot,x2dot,x3dot,x4dot,x5dot,x6dot,fx,gx] = fcn(u1,u2,x3,x4,x5,x6)

m=1;
J=0.05;
g=9.81;

x1dot = x4;
x2dot = x5;
x3dot = x6;
x4dot = -sin(x3)*u1/m;
x5dot = -g + cos(x3)*u1/m;
x6dot = u2/J;

fx = [x4;...
      x5;...
      x6;...
      0;...
      -g;...
      0];
gx = [0 0;...
      0 0;...
      0 0;...
      -sin(x3) 0;...
      cos(x3) 0;...
      0 1];

end

== matlab function A_DIOL_BicopterControl/Controlled Bicopter/Subsystem14/MATLAB Function ==
  data: x3 input; x1dot output; x4 input; x5 input; x6 input; x7 input; x8 input; x12dot output; x13dot output; x2dot output; x22dot output; x23dot output
function [x1dot,x12dot,x13dot,x2dot,x22dot,x23dot] = fcn(x3,x4,x5,x6,x7,x8)

g=9.81;
m=1;

x1dot = x4;
x12dot = -sin(x3)*x7/m;
x13dot = -cos(x3)*x6*x7/m - sin(x3)*x8/m;

x2dot = x5;
x22dot = -g + cos(x3)*x7/m;
x23dot = -sin(x3)*x6*x7/m + cos(x3)*x8/m;

end

== matlab function A_DIOL_BicopterControl/Controlled Bicopter/Subsystem15/Estimator ==
  data: xs input; gx input; u1 input; u2 input; B input; A input; Theta_hat input; Xx input; X0 input; B_dot output; A_dot output; Theta_hat_dot output; error output; Xx_dot output; X0_dot output
function [B_dot,A_dot,Theta_hat_dot,error,Xx_dot,X0_dot] = fcn(xs,gx,u1,u2,B,A,Theta_hat,Xx,X0)

theta_star = [1/1 ; 1/0.05];

%forgetting factor
lambda = 80;

%finite time
c_1 = 6;
c_2 = 3;
alpha_1 = 0.2;
alpha_2 = 1.2;

u=[u1 0;0 u2];

phi=gx*u;

%Filtered System
beta=10;
Xx_dot=-beta*Xx-beta*xs;
xf=Xx + xs;


X0_dot=-beta*X0+phi;
phif=X0;


%Finite time estimator
B_dot = phif'*phif - lambda*B;
A_dot = xf'*phif - lambda*A;
grad=Theta_hat'*B-A;
Theta_hat_dot = -c_1*grad/(norm(grad)^(1-alpha_1))-c_2*grad/(norm(grad)^(1-alpha_2));
error=norm(theta_star-Theta_hat);
end

== matlab function A_DIOL_BicopterControl/Controlled Bicopter/Subsystem15/MATLAB Function ==
  data: x input; mi output; Ji output
function [mi,Ji] = fcn(x)
mi = x(1);
Ji = x(2);
end

== matlab function A_DIOL_BicopterControl/Controlled Bicopter/Subsystem15/xsdot ==
  data: x input; xs output; intf input
function xs = fcn(x,intf)
xs = x - intf;
end

== matlab function A_DIOL_BicopterControl/Controlled Bicopter/Subsystem16/Controller ==
  data: x1r input; x1dotr input; x12dotr input; x13dotr input; x14dotr input; v1 output; x2r input; x2dotr input; x22dotr input; x23dotr input; x24dotr input; x1dot input; x12dot input; x13dot input; x2dot input; x22dot input; x23dot input; mi input; Ji input; x1 input; x2 input; x3 input; x6 input; x7 input; x8 input; v2 output; k input
function [v1,v2] = fcn(x1r,x1dotr,x12dotr,x13dotr,x14dotr,x2r,x2dotr,x22dotr,x23dotr,x24dotr,x1dot,x12dot,x13dot,x2dot,x22dot,x23dot,mi,Ji,x1,x2,x3,x6,x7,x8,k)

m = 1/mi;
J = 1/Ji;

k4 = k(1,4);
k3 = k(1,3);
k2 = k(1,2);
k1 = k(1,1);

k8 = k(2,8);
k7 = k(2,7);
k6 = k(2,6);
k5 = k(2,5);


v1 = x7*x6^2 - m*cos(x3)*(k7*(x22dot - x22dotr) - x24dotr + k8*(x23dot - x23dotr) ...
    + k5*(x2 - x2r) + k6*(x2dot - x2dotr)) + m*sin(x3)*(k3*(x12dot - x12dotr) - x14dotr ...
    + k4*(x13dot - x13dotr) + k1*(x1 - x1r) + k2*(x1dot - x1dotr));
v2 = (J*m*cos(x3)*(k3*(x12dot - x12dotr) - x14dotr + k4*(x13dot - x13dotr) ...
    + k1*(x1 - x1r) + k2*(x1dot - x1dotr)))/x7 - (2*J*x6*x8)/x7 ...
    + (J*m*sin(x3)*(k7*(x22dot - x22dotr) - x24dotr + k8*(x23dot - x23dotr) ...
    + k5*(x2 - x2r) + k6*(x2dot - x2dotr)))/x7;

end

== matlab function A_DIOL_BicopterControl/Elliptical Trajectory/r1 ==
  data: c input; r1 output; s input; r1dot output; r12dot output; r13dot output; r14dot output
function [r1,r1dot,r12dot,r13dot,r14dot] = fcn(c,s)

a1 = 5;
a2 = 3;

r1 = a1*sqrt(2)/2 - a1*sqrt(2)*c/2 - a2*sqrt(2)*s/2;
r1dot = a1*sqrt(2)*s/2 - a2*sqrt(2)*c/2;
r12dot = a1*sqrt(2)*c/2 + a2*sqrt(2)*s/2;
r13dot = -a1*sqrt(2)*s/2 + a2*sqrt(2)*c/2;
r14dot = -a1*sqrt(2)*c/2 - a2*sqrt(2)*s/2;
end

== matlab function A_DIOL_BicopterControl/Elliptical Trajectory/r2 ==
  data: c input; r1 output; s input; r1dot output; r12dot output; r13dot output; r14dot output
function [r1,r1dot,r12dot,r13dot,r14dot] = fcn(c,s)

a1 = 5;
a2 = 3;

r1 = a1*sqrt(2)/2 - a1*sqrt(2)*c/2 + a2*sqrt(2)*s/2;
r1dot = a1*sqrt(2)*s/2 + a2*sqrt(2)*c/2;
r12dot = a1*sqrt(2)*c/2 - a2*sqrt(2)*s/2;
r13dot = -a1*sqrt(2)*s/2 - a2*sqrt(2)*c/2;
r14dot = -a1*sqrt(2)*c/2 + a2*sqrt(2)*s/2;
end

== matlab function A_DIOL_BicopterControl/Controlled Bicopter 2/Subsystem1/Estimator ==
  data: xs input; gx input; u1 input; u2 input; B input; A input; Theta_hat input; Xx input; X0 input; B_dot output; A_dot output; Theta_hat_dot output; error output; Xx_dot output; X0_dot output
function [B_dot,A_dot,Theta_hat_dot,error,Xx_dot,X0_dot] = fcn(xs,gx,u1,u2,B,A,Theta_hat,Xx,X0)

theta_star = [1/1 ; 1/0.05];

%forgetting factor
lambda = 80;

%finite time
c_1 = 6;
c_2 = 3;
alpha_1 = 0.2;
alpha_2 = 1.2;

u=[u1 0;0 u2];

phi=gx*u;

%Filtered System
beta=10;
Xx_dot=-beta*Xx-beta*xs;
xf=Xx + xs;


X0_dot=-beta*X0+phi;
phif=X0;


%Finite time estimator
B_dot = phif'*phif - lambda*B;
A_dot = xf'*phif - lambda*A;
grad=Theta_hat'*B-A;
Theta_hat_dot = -c_1*grad/(norm(grad)^(1-alpha_1))-c_2*grad/(norm(grad)^(1-alpha_2));
error=norm(theta_star-Theta_hat);
end

== matlab function A_DIOL_BicopterControl/Controlled Bicopter 2/Subsystem1/MATLAB Function ==
  data: x input; mi output; Ji output
function [mi,Ji] = fcn(x)
mi = x(1);
Ji = x(2);
end

== matlab function A_DIOL_BicopterControl/Controlled Bicopter 2/Subsystem1/xsdot ==
  data: x input; xs output; intf input
function xs = fcn(x,intf)
xs = x - intf;
end

== matlab function A_DIOL_BicopterControl/Controlled Bicopter 2/Bicopter4/system ==
  data: u1 input; x1dot output; u2 input; x3 input; x4 input; x5 input; x6 input; x2dot output; x3dot output; x4dot output; x5dot output; x6dot output; fx output; gx output
function [x1dot,x2dot,x3dot,x4dot,x5dot,x6dot,fx,gx] = fcn(u1,u2,x3,x4,x5,x6)

m=1;
J=0.05;
g=9.81;

x1dot = x4;
x2dot = x5;
x3dot = x6;
x4dot = -sin(x3)*u1/m;
x5dot = -g + cos(x3)*u1/m;
x6dot = u2/J;

fx = [x4;...
      x5;...
      x6;...
      0;...
      -g;...
      0];
gx = [0 0;...
      0 0;...
      0 0;...
      -sin(x3) 0;...
      cos(x3) 0;...
      0 1];

end

== matlab function A_DIOL_BicopterControl/Controlled Bicopter 2/Subsystem11/MATLAB Function ==
  data: x3 input; x1dot output; x4 input; x5 input; x6 input; x7 input; x8 input; x12dot output; x13dot output; x2dot output; x22dot output; x23dot output
function [x1dot,x12dot,x13dot,x2dot,x22dot,x23dot] = fcn(x3,x4,x5,x6,x7,x8)

g=9.81;
m=1;

x1dot = x4;
x12dot = -sin(x3)*x7/m;
x13dot = -cos(x3)*x6*x7/m - sin(x3)*x8/m;

x2dot = x5;
x22dot = -g + cos(x3)*x7/m;
x23dot = -sin(x3)*x6*x7/m + cos(x3)*x8/m;

end
